simulink model "noisysine"  (R2020a)
settings: Solver=VariableStepAuto  StartTime=0.0  StopTime=10.0  RelTol=1e-3
libraries: dspfdesign x1
settings Model: Creator=s_moheb  LastModifiedBy=s_moheb

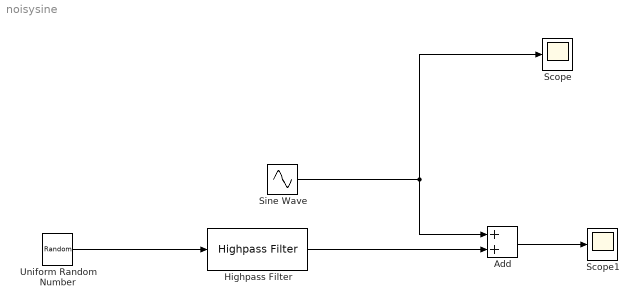
== system noisysine ==
  Add : Sum
  Highpass Filter : dspfdesign/Highpass Filter  FilterType=IIR  DesignForMinimumOrder=on  FilterOrder=50  StopbandFrequency=3600  PassbandFrequency=3800  StopbandAttenuation=60  PassbandRipple=1  InheritSampleRate=off  SampleRate=8000  SimulateUsing=Interpreted execution  roundingMode=Floor  coeffsDataTypeStr=fixdt(1,16)
  Scope : Scope
  Scope1 : Scope
  Sine Wave : Sin  Frequency=100  SampleTime=1/80000
  Uniform Random Number : UniformRandomNumber  Minimum=-5  Maximum=5  SampleTime=1/8000
  wires:
  Uniform Random Number/1 -> Highpass Filter/1
  Highpass Filter/1 -> Add/2
  Sine Wave/1 -> Scope/1, Add/1
  Add/1 -> Scope1/1
